simulink model "SistemaUchiha"  (R2024b)
settings: Solver=VariableStepAuto  StartTime=0.0  StopTime=10.0  RelTol=1e-3
settings Model: Creator=Jr  LastModifiedBy=Jr
settings DataIOCC: ReturnWorkspaceOutputs=off

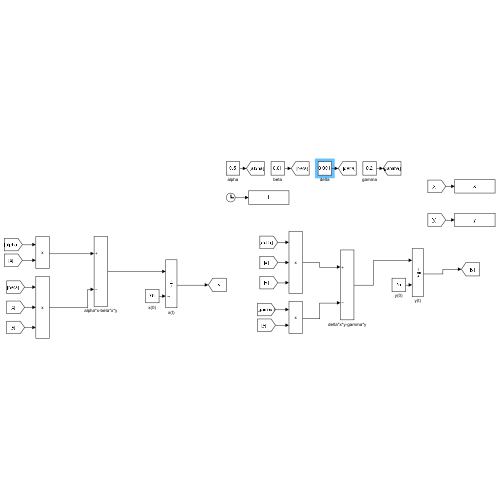
[thumbnail: Simulink's stored preview of the top-level diagram]
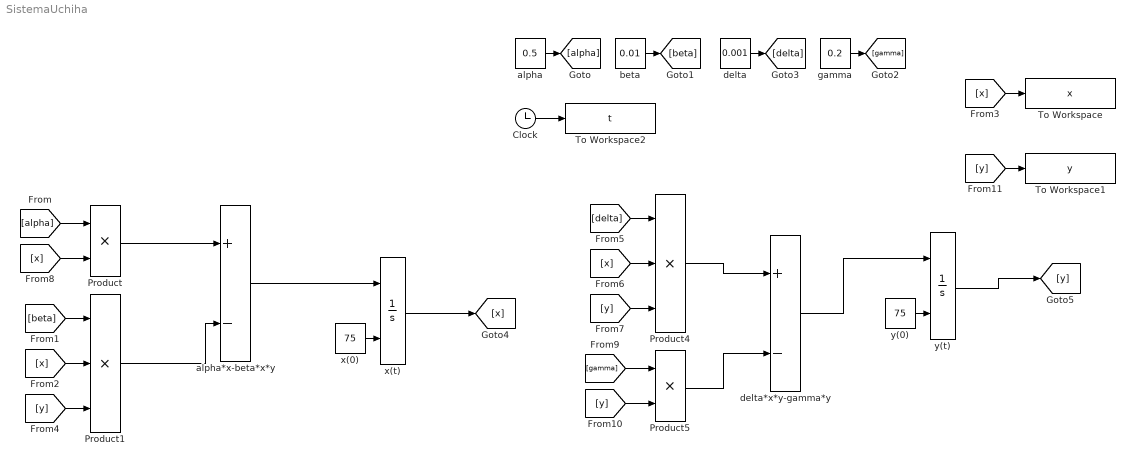
== system SistemaUchiha ==
  Clock : Clock
  Product : Product
  Product1 : Product  Inputs=3
  Product4 : Product  Inputs=3
  Product5 : Product
  To Workspace : ToWorkspace  VariableName=x  SampleTime=-1
  To Workspace1 : ToWorkspace  VariableName=y  SampleTime=-1
  To Workspace2 : ToWorkspace  VariableName=t  SampleTime=-1
  alpha : Constant  Value=0.5
  alpha*x-beta*x*y : Sum  Inputs=+-
  beta : Constant  Value=0.01
  delta : Constant  Value=0.001
  delta*x*y-gamma*y : Sum  Inputs=+-
  gamma : Constant  Value=0.2
  x(0) : Constant  Value=75
  x(t) : Integrator  InitialConditionSource=external
  y(0) : Constant  Value=75
  y(t) : Integrator  InitialConditionSource=external
  wires:
  delta*x*y-gamma*y/1 -> y(t)/1
  [x] -> Product4/2
  Product4/1 -> delta*x*y-gamma*y/1
  Product5/1 -> delta*x*y-gamma*y/2
  y(t)/1 -> [y]
  [y] -> Product4/3
  [gamma] -> Product5/1
  y(0)/1 -> y(t)/2
  [delta] -> Product4/1
  [y] -> Product5/2
  [x] -> Product/2
  Product/1 -> alpha*x-beta*x*y/1
  x(t)/1 -> [x]
  [beta] -> Product1/1
  Product1/1 -> alpha*x-beta*x*y/2
  [y] -> Product1/3
  [alpha] -> Product/1
  alpha*x-beta*x*y/1 -> x(t)/1
  [x] -> Product1/2
  x(0)/1 -> x(t)/2
  Clock/1 -> To Workspace2/1
  gamma/1 -> [gamma]
  delta/1 -> [delta]
  beta/1 -> [beta]
  alpha/1 -> [alpha]
  [y] -> To Workspace1/1
  [x] -> To Workspace/1
